simulink model "problem4_ex4"  (R2020a)
settings: Solver=VariableStepAuto  StartTime=0.0  StopTime=250  RelTol=1e-3
settings Model: Creator=dinhm  LastModifiedBy=dinhm

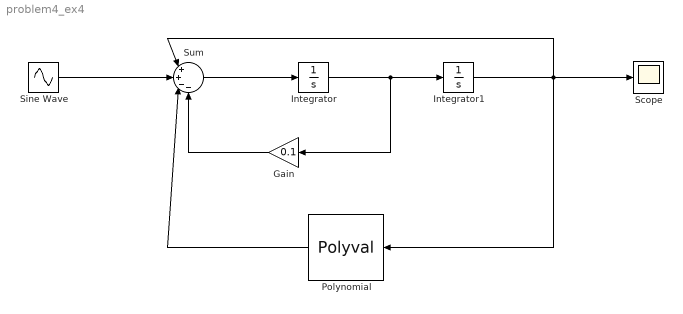
== system problem4_ex4 ==
  Gain : Gain  Gain=0.1
  Integrator : Integrator  InitialCondition=0.29
  Integrator1 : Integrator  InitialCondition=0.585
  Polynomial : Polyval  Coefs=[1,0,0,0]
  Scope : Scope
  Sine Wave : Sin  Amplitude=0.07  Frequency=1.25  Phase=pi/2  SampleTime=0
  Sum : Sum  Inputs=|++--
  wires:
  Sine Wave/1 -> Sum/2
  Gain/1 -> Sum/4
  Sum/1 -> Integrator/1
  Integrator/1 -> Gain/1, Integrator1/1
  Integrator1/1 -> Sum/1, Polynomial/1, Scope/1
  Polynomial/1 -> Sum/3
